simulink model "dspAudioPos"  (Simulink 8.3)
settings: Solver=FixedStepDiscrete  StartTime=0.0  StopTime=60  RelTol=1e-3
model workspace (MAT data in the model file):
  heli = [0 -3.0517578125e-05 -0.0001220703125 -0.000244140625 -0.0003662109375 -0.000701904296875 -0.00106811523438 -0.00204467773438 -0.00341796875 -0.00460815429688 -0.00595092773438 -0.00762939453125 ... (263304 elements, 263304x1)]
  h : num (value not decoded)
libraries: dspsrcs4 x1, dspmisc x1, dspsnks4 x1
CloseFcn:
  | try
  |     h = evalin(get_param(gcs, 'ModelWorkspace'), 'h');
  |     close(h);
  | catch
  | end
settings Model: Creator=The MathWorks Inc.
settings OptimizationCC: ExpressionDepthLimit=2147483647  RollThreshold=1  InitFltsAndDblsToZero=on  EfficientMapNaN2IntZero=off
settings DebuggingCC: SolverPrmCheckMsg=none  InheritedTsInSrcMsg=none  FcnCallInpInsideContextMsg=UseLocalSettings  StrictBusMsg=Warning
settings SFSimCC: SimParseCustomCode=off

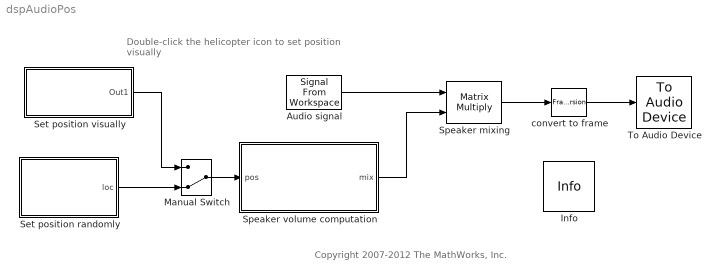
== system dspAudioPos ==
  note: Double-click the helicopter icon
      | to set position visually
  note: Copyright 2007-2012 The MathWorks, Inc.
  " Set position visually" : Subsystem  mask{loc=[0.591818181818182 0.735454545454545]}
      mask init:
      | I = imread('helicopter.jpg');
      settings: OpenFcn=assignin(get_param(gcs, 'ModelWorkspace'), 'h', dspAudioPosGui(str2num(get_param(gcb,'loc')), gcb, @(blk,loc)(set_param(blk,'loc',loc))));
      mask Display: image(I);
  Audio signal : dspsrcs4/Signal From Workspace  X=heli  Ts=1/44100  nsamps=1024  OutputAfterFinalValue=Cyclic repetition  ignoreOrWarnInputAndFrameLengths=off
  Info : dspmisc/Info  SystemSampleTime=-1
  Manual Switch : ManualSwitch  CurrentSetting=0
  Set position randomly : MATLAB Function  TreatAsAtomicUnit=on
  Speaker mixing : Product  Multiplication=Matrix(*)
  Speaker volume computation : MATLAB Function  TreatAsAtomicUnit=on
  To Audio Device : dspsnks4/To Audio Device  deviceName=Default  inheritSampleRate=on  sampleRate=44100  deviceDatatype=16-bit integer  autoBufferSize=off  bufferSize=1024  queueDuration=2  defaultOutputChannelMapping=on  outputChannelMapping=1
  "convert to frame " : FrameConversion
  wires:
  Speaker mixing/1 -> "convert to frame "/1
  "convert to frame "/1 -> To Audio Device/1
  Speaker volume computation/1(mix) -> Speaker mixing/2
  " Set position visually"/1(Out1) -> Manual Switch/1
  Manual Switch/1 -> Speaker volume computation/1(pos)
  Set position randomly/1(loc) -> Manual Switch/2
  Audio signal/1 -> Speaker mixing/1

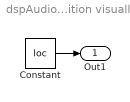
== system dspAudioPos/ Set position visually ==
  Constant : Constant  Value=loc  VectorParams1D=off  SampleTime=-1
  Out1 : Outport
  wires:
  Constant/1 -> Out1/1

== matlab function Set position randomly ==
  data: loc output double
function loc = randomLoc()
% This block Computes a random position in a unit circle. 

persistent lastLoc;

if isempty(lastLoc)
    lastLoc = [0 0.5];
end

lastLoc = lastLoc + 0.02*randn(1,2);
nrm = norm(lastLoc);
if nrm > 1
    lastLoc = lastLoc / nrm;
end
loc = lastLoc;

== matlab function Speaker volume computation ==
  data: pos input double; mix output double
function mix = computeVol(pos)
% This block Computes a speaker mixing matrix based on
% the source location. 

% left front
% right front
% front center
% low frequency
% left rear
% right rear

% x,y speaker locations
speakerLoc = [-1 1; 1 1; 0 sqrt(2); -1 -1; 1 -1] ./ sqrt(2);

sourceDistance = norm(pos);
sourceDir      = pos / sourceDistance;

amp = 0.5 * (speakerLoc * pos');
[dist ndx] = sort(amp, 'descend');
sideMix = [0 0 0 0 0];

% Determine the vector of speaker amplitudes
if sourceDistance == 0
    % They are dead center.
% Can we represent the sound with one speaker?
elseif amp(ndx(1)) == sourceDistance
    sideMix(ndx(1)) = 1;
    
% OK, split the sound between speakers.
else
    % Find the closest vector.
    closest = ndx(1:2);
    % The second 'closest' vector is the closest vector to the source 
    % which is further away from the closest vector.
    for i=2:length(ndx)
        if speakerLoc(closest(1),:) * speakerLoc(ndx(i),:)' > ...
           sourceDir * speakerLoc(ndx(i),:)'
           closest(2) = ndx(i+1);
        else
            break;
        end
    end
    % Express the source direction using the nearest two speaker vectors
    % as a basis
    p = sourceDir;
    L = speakerLoc(closest, :);
    g = p * inv(L);
    % Re-normalize.
    % This is really only necessary for the center channel.
    g = g/norm(g);
    sideMix(closest) = g;
end


% We computed the balance as if the source were on the unit circle.
% In the middle of the cirle, this algorithm will produce an effect 
% which is too "discrete".  Hence, we will cross-fade to the outer ring 
% from a center where we assume that all speakers are on.
 

% Set all speaker amplitudes equal when in the center.
centerMix = repmat(1, [1 6]);

% Mix from the center to the side allocation strategy, and then normalize 
% the power so that it remains constant.
mix = centerMix*centerFalloff(sourceDistance) +...
    + [sideMix(1:3) 0 sideMix(4:5)]*(1-centerFalloff(sourceDistance) );
mix = mix / norm(mix);

% Finally, adjust the amplitude so that it falls off with an inverse 
% square law, and the perimeter is 1/4 as loud as the center.  Since we 
% know that the maximum amplitude of a channel is 1/sqrt(6) (which happens 
% in the center), we multiply by sqrt(6). 
mix = sqrt(6) * mix * (1/(1+sourceDistance))^2;
end


function amp = centerFalloff(sourceDistance)
    amp = (1-sourceDistance)^2;
end
